simulink model "Model_6DOF_B3_2019a"  (R2019a)
settings: Solver=FixedStepAuto  StartTime=0.0  StopTime=200  FixedStep=0.05  RelTol=1e-3
values from neighbouring files (symbols this model uses):
  Ba_0 = [0 0 0 0 0 0]    [ctrl_mode_param.m]
  Bb = 4418825.3321    [load_data.m]
  Bv_0 = [tgt_speed 0 0 0 0 0]    [ctrl_mode_param.m]
  Bx_0 = [0 0 tgt_depth 0 0 0]    [ctrl_mode_param.m]
  check_angle = 10    [ctrl_mode_param.m]
  dX_imposed = 10    [ctrl_mode_param.m]
  Ixx = 5.23e7    (= 52300000)    [load_data.m]
  Ixy = 0    [load_data.m]
  Ixz = 0    [load_data.m]
  Iyy = 1.375e9    (= 1375000000)    [load_data.m]
  Iyz = 0    [load_data.m]
  Izz = 1.367e9    (= 1367000000)    [load_data.m]
  Mb = 4418825.3321    [load_data.m]
  Seastate = 5    [ctrl_mode_param.m]    (also in run.m = 0)
  Xb = 0    [load_data.m]
  Xg = 0    [load_data.m]
  Yb = 0    [load_data.m]
  Yg = 0    [load_data.m]
  Zb = 0.4406    [load_data.m]
  Zg = 0    [load_data.m]
undefined symbols (not defined in the file or in its folder): dA_BP1, dA_BP2, dA_Hull, dA_PH, dA_Sail, dA_SProot, dA_X1a, dA_X1b, dA_X2a, dA_X2b, dA_X3a, dA_X3b, dA_X4a, dA_X4b, DoF_switch, fwrite, its, LCG_switch, m_switch, mass_switch, n_BP1, n_BP2, n_Hull, n_imposed, n_PH, n_Sail, n_SProot, n_switch, n_X1a, n_X1b, n_X2a, n_X2b, n_X3a, n_X3b, n_X4a, n_X4b, nt_BP1, nt_BP2, nt_Hull, nt_PH, nt_Sail, nt_SProot, nt_X1a, nt_X1b, nt_X2a, nt_X2b, nt_X3a, nt_X3b, nt_X4a, nt_X4b, sail_switch, target_pitch, target_y, target_yaw, target_z, Usp, vt1_BP1, vt1_BP2, vt1_Hull, vt1_PH ... (+38)
libraries: simulink x5
(part 1 of 6)
settings Model: OrderedModelArguments=off  Creator=yagkim  LastModifiedBy=cooki
settings DebuggingCC: UnderSpecifiedDimensionMsg=warning

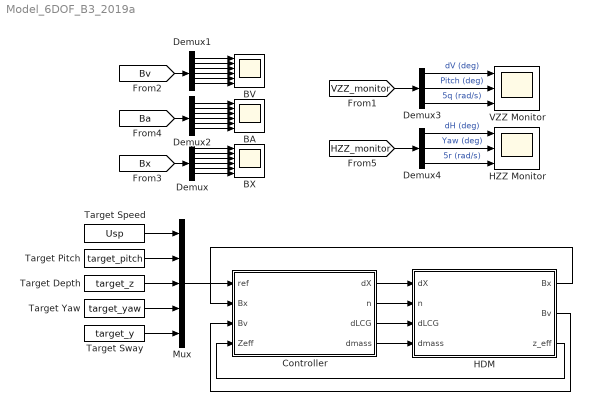
== system Model_6DOF_B3_2019a ==
  BA : Scope  NumInputPorts=6
  BV : Scope  NumInputPorts=6
  BX : Scope  NumInputPorts=6
  Controller : Subsystem
  Demux : Demux  Outputs=6
  Demux1 : Demux  Outputs=6
  Demux2 : Demux  Outputs=6
  Demux3 : Demux  Outputs=3
  Demux4 : Demux  Outputs=3
  HDM : Subsystem
  HZZ Monitor : Scope  NumInputPorts=3
  Mux : Mux  Inputs=5
  Target Depth : Constant  Value=target_z
  Target Pitch : Constant  Value=target_pitch
  Target Speed : Constant  Value=Usp
  Target Sway : Constant  Value=target_y
  Target Yaw : Constant  Value=target_yaw
  VZZ Monitor : Scope  NumInputPorts=3
  wires:
  Demux/1 -> BX/1
  Demux/2 -> BX/2
  Demux/3 -> BX/3
  Demux/6 -> BX/6
  Mux/1 -> Controller/1(ref)
  Target Speed/1 -> Mux/1
  Target Depth/1 -> Mux/3
  Demux/5 -> BX/5
  Demux2/4 -> BA/4
  Demux2/1 -> BA/1
  Demux2/3 -> BA/3
  Demux2/6 -> BA/6
  Demux2/5 -> BA/5
  Demux2/2 -> BA/2
  Target Pitch/1 -> Mux/2
  Target Yaw/1 -> Mux/4
  Target Sway/1 -> Mux/5
  Demux1/4 -> BV/4
  Demux1/6 -> BV/6
  Demux1/1 -> BV/1
  Demux1/2 -> BV/2
  Demux1/3 -> BV/3
  Demux1/5 -> BV/5
  [Bv] -> Demux1/1
  [Ba] -> Demux2/1
  [Bx] -> Demux/1
  HDM/1(Bx) -> Controller/2(Bx)
  HDM/2(Bv) -> Controller/3(Bv)
  Controller/1(dX) -> HDM/1(dX)
  Controller/2(n) -> HDM/2(n)
  Controller/3(dLCG) -> HDM/3(dLCG)
  Controller/4(dmass) -> HDM/4(dmass)
  HDM/3(z_eff) -> Controller/4(Zeff)
  Demux4/2 -> HZZ Monitor/2  "Yaw (deg)"
  [VZZ_monitor] -> Demux3/1
  Demux3/3 -> VZZ Monitor/3  "5q (rad/s)"
  Demux4/3 -> HZZ Monitor/3  "5r (rad/s)"
  Demux3/1 -> VZZ Monitor/1  "dV (deg)"
  Demux4/1 -> HZZ Monitor/1  "dH (deg)"
  [HZZ_monitor] -> Demux4/1
  Demux3/2 -> VZZ Monitor/2  "Pitch (deg)"
  Demux/4 -> BX/4

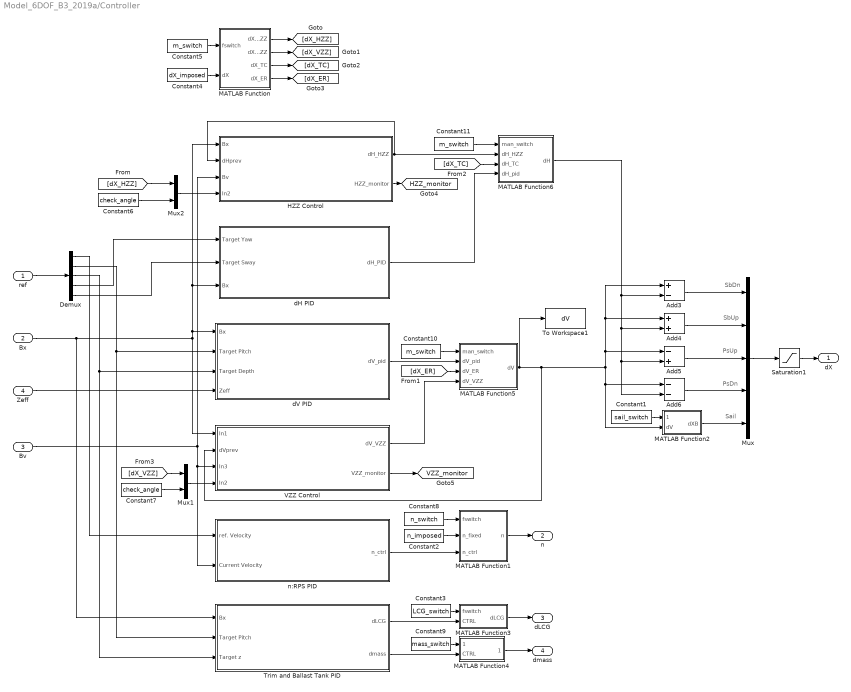
== system Model_6DOF_B3_2019a/Controller ==
  note: SbDn
  note: SbUp
  note: PsUp
  note: PsDn
  note: Sail
  ref : Inport
  Bx : Inport  Port=2
  Bv : Inport  Port=3
  Zeff : Inport  Port=4
  Add3 : Sum  Inputs=+-
  Add4 : Sum
  Add5 : Sum  Inputs=-+
  Add6 : Sum  Inputs=--
  Constant1 : Constant  Value=sail_switch
  Constant10 : Constant  Value=m_switch
  Constant11 : Constant  Value=m_switch
  Constant2 : Constant  Value=n_imposed
  Constant3 : Constant  Value=LCG_switch
  Constant4 : Constant  Value=dX_imposed
  Constant5 : Constant  Value=m_switch
  Constant6 : Constant  Value=check_angle
  Constant7 : Constant  Value=check_angle
  Constant8 : Constant  Value=n_switch
  Constant9 : Constant  Value=mass_switch
  Demux : Demux  Outputs=5
  HZZ Control : Subsystem
  MATLAB Function : MATLAB Function  TreatAsAtomicUnit=on
  MATLAB Function1 : MATLAB Function  TreatAsAtomicUnit=on
  MATLAB Function2 : MATLAB Function  TreatAsAtomicUnit=on
  MATLAB Function3 : MATLAB Function  TreatAsAtomicUnit=on
  MATLAB Function4 : MATLAB Function  TreatAsAtomicUnit=on
  MATLAB Function5 : MATLAB Function  TreatAsAtomicUnit=on
  MATLAB Function6 : MATLAB Function  TreatAsAtomicUnit=on
  Mux : Mux  Inputs=5
  Mux1 : Mux  Inputs=2
  Mux2 : Mux  Inputs=2
  Saturation1 : Saturate  UpperLimit=30  LowerLimit=-30
  To Workspace1 : ToWorkspace  VariableName=dV  SaveFormat=Timeseries  SampleTime=-1
  Trim and Ballast Tank PID : Subsystem
  VZZ Control : Subsystem
  dH PID : Subsystem
  dV PID : Subsystem
  n:RPS PID : Subsystem
  dX : Outport  VectorParamsAs1DForOutWhenUnconnected=off
  n : Outport  Port=2  VectorParamsAs1DForOutWhenUnconnected=off
  dLCG : Outport  Port=3  VectorParamsAs1DForOutWhenUnconnected=off
  dmass : Outport  Port=4  VectorParamsAs1DForOutWhenUnconnected=off
  tag scope: HZZ_monitor=global, VZZ_monitor=global
  wires:
  Add3/1 -> Mux/1
  Add4/1 -> Mux/2
  Add5/1 -> Mux/3
  Add6/1 -> Mux/4
  MATLAB Function2/1(dXB) -> Mux/5
  MATLAB Function5/1(dV) -> To Workspace1/1, VZZ Control/2(dVprev), Add3/1, Add4/1, Add5/1, MATLAB Function2/2(dV), Add6/1
  Bv/1 -> HZZ Control/3(Bv), n:RPS PID/2(Current Velocity), VZZ Control/3(In3)
  Demux/1 -> n:RPS PID/1(ref. Velocity)
  n:RPS PID/1(n_ctrl) -> MATLAB Function1/3(n_ctrl)
  ref/1 -> Demux/1
  dV PID/1(dV_pid) -> MATLAB Function5/2(dV_pid)
  Demux/4 -> dH PID/1(Target Yaw)
  Demux/5 -> dH PID/2(Target Sway)
  Mux1/1 -> VZZ Control/4(In2)
  [dX_VZZ] -> Mux1/1
  Constant7/1 -> Mux1/2
  Demux/2 -> Trim and Ballast Tank PID/2(Target Pitch), dV PID/2(Target Pitch)
  Bx/1 -> Trim and Ballast Tank PID/1(Bx), HZZ Control/1(Bx), dH PID/3(Bx), dV PID/1(Bx), VZZ Control/1(In1)
  Demux/3 -> Trim and Ballast Tank PID/3(Target z), dV PID/3(Target Depth)
  MATLAB Function3/1(dLCG) -> dLCG/1
  Mux/1 -> Saturation1/1
  Constant6/1 -> Mux2/2
  Mux2/1 -> HZZ Control/4(In2)
  [dX_HZZ] -> Mux2/1
  MATLAB Function6/1(dH) -> Add6/2, Add5/2, Add4/2, Add3/2
  Zeff/1 -> dV PID/4(Zeff)
  Saturation1/1 -> dX/1
  MATLAB Function4/1(dmass) -> dmass/1
  Constant5/1 -> MATLAB Function/1(fswitch)
  Constant4/1 -> MATLAB Function/2(dX)
  MATLAB Function/1(dX_HZZ) -> [dX_HZZ]
  MATLAB Function/2(dX_VZZ) -> [dX_VZZ]
  MATLAB Function/3(dX_TC) -> [dX_TC]
  MATLAB Function/4(dX_ER) -> [dX_ER]
  Constant8/1 -> MATLAB Function1/1(fswitch)
  Constant2/1 -> MATLAB Function1/2(n_fixed)
  MATLAB Function1/1(n) -> n/1
  Constant1/1 -> MATLAB Function2/1(fswitch)
  VZZ Control/2(VZZ_monitor) -> [VZZ_monitor]
  Trim and Ballast Tank PID/1(dLCG) -> MATLAB Function3/2(CTRL)
  Constant3/1 -> MATLAB Function3/1(fswitch)
  Trim and Ballast Tank PID/2(dmass) -> MATLAB Function4/2(CTRL)
  Constant9/1 -> MATLAB Function4/1(fswitch)
  [dX_TC] -> MATLAB Function6/3(dH_TC)
  Constant10/1 -> MATLAB Function5/1(man_switch)
  [dX_ER] -> MATLAB Function5/3(dV_ER)
  VZZ Control/1(dV_VZZ) -> MATLAB Function5/4(dV_VZZ)
  Constant11/1 -> MATLAB Function6/1(man_switch)
  HZZ Control/1(dH_HZZ) -> HZZ Control/2(dHprev), MATLAB Function6/2(dH_HZZ)
  dH PID/1(dH_PID) -> MATLAB Function6/4(dH_pid)
  HZZ Control/2(HZZ_monitor) -> [HZZ_monitor]

== system Model_6DOF_B3_2019a/HDM ==
  dX : Inport
  n : Inport  Port=2
  dLCG : Inport  Port=3
  dmass : Inport  Port=4
  Constant : Constant  Value=fwrite
  Constant1 : Constant  Value=Seastate
  HDM B3 : Subsystem  InitFcn='main'
  Integration and Coord. Transfrom : Subsystem
  Bx : Outport
  Bv : Outport  Port=2
  z_eff : Outport  Port=3
  tag scope: Ba=global, Bv=global, Bx=global
  wires:
  dLCG/1 -> HDM B3/3(dLCG)
  n/1 -> HDM B3/2(n)
  Integration and Coord. Transfrom/1(Bas) -> [Ba], HDM B3/7(Ba)
  dX/1 -> HDM B3/1(dX CTRL)
  dmass/1 -> HDM B3/4(dmass)
  HDM B3/2(z_eff) -> z_eff/1
  Integration and Coord. Transfrom/3(Bv) -> HDM B3/6(Bv), Bv/1, [Bv]
  HDM B3/1(F_hyd) -> Integration and Coord. Transfrom/2(F_hyd)
  Constant1/1 -> HDM B3/9(SeaState)
  Constant/1 -> HDM B3/8(fwrite)
  Integration and Coord. Transfrom/2("Bx ") -> Integration and Coord. Transfrom/1(Bx), HDM B3/5(Bx), Bx/1, [Bx]

== system Model_6DOF_B3_2019a/Controller/HZZ Control ==
  Bx : Inport
  dHprev : Inport  Port=2
  Bv : Inport  Port=3
  In2 : Inport  Port=4
  Clock : Clock
  Demux : Demux  Outputs=2
  Gain1 : Gain  Gain=-1
  Gain10 : Gain  Gain=180/pi
  Gain11 : Gain  Gain=5
  Gain3 : Gain
  Gain4 : Gain
  Gain8 : Gain  Gain=180/pi
  Integrator2 : Integrator
  MATLAB Function : MATLAB Function  TreatAsAtomicUnit=on
  Max Fin Rate : Constant  Value=7.11
  Mux2 : Mux  Inputs=3
  Saturation4 : Saturate  UpperLimit=20  LowerLimit=-20
  Scope : Scope
  Selector2 : Selector  InputPortWidth=6  IndexOptions=Index vector (dialog)  Indices=6  OutputSizes=1
  Selector3 : Selector  InputPortWidth=6  IndexOptions=Index vector (dialog)  Indices=6  OutputSizes=1
  dH_HZZ : Outport
  HZZ_monitor : Outport  Port=2
  wires:
  Gain11/1 -> Mux2/3
  Selector3/1 -> Gain10/1
  MATLAB Function/1(dVrate) -> Integrator2/1
  Gain10/1 -> Gain11/1
  Max Fin Rate/1 -> MATLAB Function/1(rate)
  Selector2/1 -> Gain8/1
  Clock/1 -> MATLAB Function/2(trigger)
  Gain8/1 -> Gain3/1
  Bx/1 -> Selector2/1
  Integrator2/1 -> Saturation4/1
  Saturation4/1 -> MATLAB Function/4(dVprev), Gain1/1
  Bv/1 -> Selector3/1
  Mux2/1 -> HZZ_monitor/1
  In2/1 -> Gain4/1
  Demux/1 -> MATLAB Function/5(dVmax)
  Demux/2 -> MATLAB Function/6(dXmax)
  Gain1/1 -> Scope/1, dH_HZZ/1
  Gain4/1 -> Demux/1
  Gain3/1 -> Mux2/2, MATLAB Function/3(X5)
  dHprev/1 -> Mux2/1

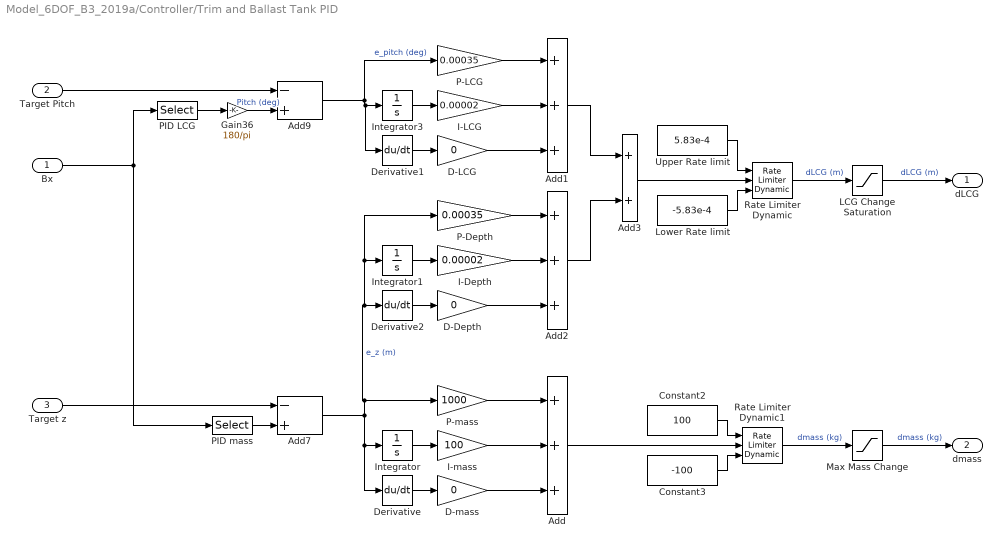
== system Model_6DOF_B3_2019a/Controller/Trim and Ballast Tank PID ==
  Bx : Inport
  Target Pitch : Inport  Port=2
  Target z : Inport  Port=3
  " LCG Change Saturation" : Saturate
  Add : Sum  Inputs=+++
  Add1 : Sum  Inputs=+++
  Add2 : Sum  Inputs=+++
  Add3 : Sum
  Add7 : Sum  Inputs=-+
  Add9 : Sum  Inputs=-+
  Constant2 : Constant  Value=100
  Constant3 : Constant  Value=-100
  D-Depth : Gain  Gain=0
  D-LCG : Gain  Gain=0
  D-mass : Gain  Gain=0
  Derivative : Derivative
  Derivative1 : Derivative
  Derivative2 : Derivative
  Gain36 : Gain  Gain=180/pi
  I-Depth : Gain  Gain=0.00002
  I-LCG : Gain  Gain=0.00002
  I-mass : Gain  Gain=100
  Integrator : Integrator
  Integrator1 : Integrator
  Integrator3 : Integrator
  Lower Rate limit : Constant  Value=-5.83e-4
  Max Mass Change : Saturate  UpperLimit=20000  LowerLimit=-20000
  P-Depth : Gain  Gain=0.00035
  P-LCG : Gain  Gain=0.00035
  P-mass : Gain  Gain=1000
  PID LCG : Selector  InputPortWidth=6  IndexOptions=Index vector (dialog)  Indices=5  OutputSizes=1
  PID mass : Selector  InputPortWidth=6  IndexOptions=Index vector (dialog)  Indices=3  OutputSizes=1
  Rate Limiter Dynamic : simulink/Discontinuities/Rate Limiter Dynamic
  Rate Limiter Dynamic1 : simulink/Discontinuities/Rate Limiter Dynamic
  Upper Rate limit : Constant  Value=5.83e-4
  dLCG : Outport
  dmass : Outport  Port=2
  wires:
  D-mass/1 -> Add/3
  Bx/1 -> PID LCG/1, PID mass/1
  I-mass/1 -> Add/2
  Gain36/1 -> Add9/2  "Pitch (deg)"
  P-LCG/1 -> Add1/1
  D-LCG/1 -> Add1/3
  PID LCG/1 -> Gain36/1
  Rate Limiter Dynamic/1 -> " LCG Change Saturation"/1  "dLCG (m)"
  Integrator/1 -> I-mass/1
  Target z/1 -> Add7/1
  Derivative/1 -> D-mass/1
  PID mass/1 -> Add7/2
  Derivative1/1 -> D-LCG/1
  Integrator3/1 -> I-LCG/1
  I-LCG/1 -> Add1/2
  P-mass/1 -> Add/1
  Target Pitch/1 -> Add9/1
  Upper Rate limit/1 -> Rate Limiter Dynamic/1
  Lower Rate limit/1 -> Rate Limiter Dynamic/3
  Max Mass Change/1 -> dmass/1  "dmass (kg)"
  Add/1 -> Rate Limiter Dynamic1/2
  Rate Limiter Dynamic1/1 -> Max Mass Change/1  "dmass (kg)"
  Constant2/1 -> Rate Limiter Dynamic1/1
  Constant3/1 -> Rate Limiter Dynamic1/3
  " LCG Change Saturation"/1 -> dLCG/1  "dLCG (m)"
  I-Depth/1 -> Add2/2
  Integrator1/1 -> I-Depth/1
  Derivative2/1 -> D-Depth/1
  D-Depth/1 -> Add2/3
  P-Depth/1 -> Add2/1
  Add3/1 -> Rate Limiter Dynamic/2
  Add1/1 -> Add3/1
  Add2/1 -> Add3/2
  Add7/1 -> Derivative/1, Integrator/1, P-Depth/1, Integrator1/1, Derivative2/1, P-mass/1  "e_z (m)"
  Add9/1 -> Derivative1/1, Integrator3/1, P-LCG/1  "e_pitch (deg)"

== system Model_6DOF_B3_2019a/Controller/VZZ Control ==
  In1 : Inport
  dVprev : Inport  Port=2
  In3 : Inport  Port=3
  In2 : Inport  Port=4
  Clock : Clock
  Demux : Demux  Outputs=2
  Gain1 : Gain  Gain=-1
  Gain10 : Gain  Gain=180/pi
  Gain11 : Gain  Gain=5
  Gain8 : Gain  Gain=180/pi
  Integrator2 : Integrator
  MATLAB Function : MATLAB Function  TreatAsAtomicUnit=on
  Max Fin Rate : Constant  Value=7.11
  Mux2 : Mux  Inputs=3
  Saturation4 : Saturate  UpperLimit=20  LowerLimit=-20
  Selector2 : Selector  InputPortWidth=6  IndexOptions=Index vector (dialog)  Indices=5  OutputSizes=1
  Selector3 : Selector  InputPortWidth=6  IndexOptions=Index vector (dialog)  Indices=5  OutputSizes=1
  dV_VZZ : Outport
  VZZ_monitor : Outport  Port=2
  wires:
  Gain11/1 -> Mux2/3
  Selector3/1 -> Gain10/1
  MATLAB Function/1(dVrate) -> Integrator2/1
  Gain10/1 -> Gain11/1
  Max Fin Rate/1 -> MATLAB Function/1(rate)
  dVprev/1 -> Mux2/1
  Selector2/1 -> Gain8/1
  Clock/1 -> MATLAB Function/2(trigger)
  Gain8/1 -> MATLAB Function/3(X5), Mux2/2
  In1/1 -> Selector2/1
  Integrator2/1 -> Saturation4/1
  Saturation4/1 -> MATLAB Function/4(dVprev), Gain1/1
  In3/1 -> Selector3/1
  Mux2/1 -> VZZ_monitor/1
  In2/1 -> Demux/1
  Demux/1 -> MATLAB Function/5(dVmax)
  Demux/2 -> MATLAB Function/6(dXmax)
  Gain1/1 -> dV_VZZ/1

== system Model_6DOF_B3_2019a/Controller/dH PID ==
  Target Yaw : Inport
  Target Sway : Inport  Port=2
  Bx : Inport  Port=3
  Add1 : Sum  Inputs=+++
  Add10 : Sum
  Add2 : Sum  Inputs=+++
  Add7 : Sum  Inputs=-+
  Add9 : Sum  Inputs=-+
  Constant : Constant  Value=7.11
  Constant1 : Constant  Value=-7.11
  D-Sway : Gain  Gain=0
  D-Yaw : Gain  Gain=12.199
  Derivative : Derivative
  Derivative1 : Derivative
  Gain36 : Gain  Gain=180/pi
  I-Sway : Gain  Gain=0
  I-Yaw : Gain  Gain=0
  Integrator : Integrator
  Integrator3 : Integrator
  Max Deflection : Saturate  UpperLimit=30  LowerLimit=-30
  P-Sway1 : Gain  Gain=-1.452
  P-Yaw : Gain  Gain=3
  PID Sway : Selector  InputPortWidth=6  IndexOptions=Index vector (dialog)  Indices=2  OutputSizes=1
  PID Yaw : Selector  InputPortWidth=6  IndexOptions=Index vector (dialog)  Indices=6  OutputSizes=1
  Rate Limiter Dynamic : simulink/Discontinuities/Rate Limiter Dynamic
  dH_PID : Outport
  wires:
  Integrator3/1 -> I-Yaw/1
  Add9/1 -> P-Yaw/1, Derivative1/1, Integrator3/1
  Add2/1 -> Add10/2
  I-Yaw/1 -> Add1/2
  Add7/1 -> P-Sway1/1, Derivative/1, Integrator/1
  Target Sway/1 -> Add7/1
  Derivative/1 -> D-Sway/1
  PID Sway/1 -> Add7/2
  P-Yaw/1 -> Add1/1
  Bx/1 -> PID Yaw/1, PID Sway/1
  I-Sway/1 -> Add2/2
  Rate Limiter Dynamic/1 -> Max Deflection/1
  D-Yaw/1 -> Add1/3
  PID Yaw/1 -> Gain36/1
  Add1/1 -> Add10/1
  Integrator/1 -> I-Sway/1
  Gain36/1 -> Add9/2
  Max Deflection/1 -> dH_PID/1
  P-Sway1/1 -> Add2/1
  D-Sway/1 -> Add2/3
  Derivative1/1 -> D-Yaw/1
  Add10/1 -> Rate Limiter Dynamic/2
  Target Yaw/1 -> Add9/1
  Constant1/1 -> Rate Limiter Dynamic/3
  Constant/1 -> Rate Limiter Dynamic/1

== system Model_6DOF_B3_2019a/Controller/dV PID ==
  Bx : Inport
  Target Pitch : Inport  Port=2
  Target Depth : Inport  Port=3
  Zeff : Inport  Port=4
  Add : Sum  Inputs=+++
  Add1 : Sum  Inputs=+++
  Add10 : Sum
  Add7 : Sum  Inputs=-+
  Add9 : Sum  Inputs=-+
  Constant : Constant  Value=7.11
  Constant1 : Constant  Value=-7.11
  D-Depth : Gain  Gain=3
  D-Pitch : Gain  Gain=3
  Derivative : Derivative
  Derivative3 : Derivative
  Gain36 : Gain  Gain=180/pi
  I-Depth : Gain  Gain=0.1044
  I-Pitch : Gain  Gain=0.1466
  I-Pitch{1..6} (6 alike) : Gain
  Integrator : Integrator
  Integrator3 : Integrator
  Max Deflection : Saturate  UpperLimit=30  LowerLimit=-30
  P-Depth : Gain  Gain=3
  P-Pitch : Gain  Gain=3
  PID Pitch : Selector  InputPortWidth=6  IndexOptions=Index vector (dialog)  Indices=5  OutputSizes=1
  Rate Limiter Dynamic : simulink/Discontinuities/Rate Limiter Dynamic
  dV_pid : Outport
  wires:
  Add/1 -> Add10/2  "dV Depth (deg)"
  Add7/1 -> Derivative3/1, Integrator/1, P-Depth/1  "Erorr in z (m)"
  Zeff/1 -> Add7/2  "z (m)"
  Integrator/1 -> I-Depth/1
  P-Depth/1 -> I-Pitch4/1
  Gain36/1 -> Add9/2  "Pitch (deg)"
  Add9/1 -> Derivative/1, Integrator3/1, P-Pitch/1  "Error in Pitch (deg)"
  P-Pitch/1 -> I-Pitch3/1
  Bx/1 -> PID Pitch/1
  Derivative3/1 -> D-Depth/1
  Add1/1 -> Add10/1  "dV Pitch (deg)"
  D-Depth/1 -> I-Pitch6/1
  Derivative/1 -> D-Pitch/1
  Integrator3/1 -> I-Pitch/1
  PID Pitch/1 -> Gain36/1
  Max Deflection/1 -> dV_pid/1  "dV"
  D-Pitch/1 -> I-Pitch5/1
  Target Pitch/1 -> Add9/1
  Add10/1 -> Rate Limiter Dynamic/2
  Rate Limiter Dynamic/1 -> Max Deflection/1
  Constant/1 -> Rate Limiter Dynamic/1
  Constant1/1 -> Rate Limiter Dynamic/3
  Target Depth/1 -> Add7/1
  I-Pitch/1 -> I-Pitch1/1
  I-Depth/1 -> I-Pitch2/1
  I-Pitch1/1 -> Add1/2
  I-Pitch2/1 -> Add/2
  I-Pitch3/1 -> Add1/1
  I-Pitch4/1 -> Add/1
  I-Pitch5/1 -> Add1/3
  I-Pitch6/1 -> Add/3

== system Model_6DOF_B3_2019a/Controller/n:RPS PID ==
  ref. Velocity : Inport
  Current Velocity : Inport  Port=2
  Add : Sum  Inputs=+++
  Add1 : Sum  Inputs=-+
  Constant1 : Constant  Value=4
  Divide : Product  Inputs=*/
  Gain1 : Gain  Gain=14.65
  Gain4 : Gain  Gain=1.465
  Integrator : Integrator
  Rate Limiter Dynamic : simulink/Discontinuities/Rate Limiter Dynamic
  Rate Max : Constant  Value=14.65
  Rate Min : Constant  Value=-14.65
  Saturation6 : Saturate  UpperLimit=10  LowerLimit=0.01
  Selector : Selector  InputPortWidth=6  IndexOptions=Index vector (dialog)  Indices=1  OutputSizes=1
  n_ctrl : Outport  VectorParamsAs1DForOutWhenUnconnected=off
  wires:
  Selector/1 -> Add1/2  "current"
  Constant1/1 -> Divide/2
  ref. Velocity/1 -> Add1/1, Divide/1  "target"
  Add1/1 -> Gain1/1, Integrator/1  "error term"
  Current Velocity/1 -> Selector/1
  Gain4/1 -> Add/3
  Gain1/1 -> Add/2
  Add/1 -> Rate Limiter Dynamic/2
  Divide/1 -> Add/1
  Rate Limiter Dynamic/1 -> Saturation6/1
  Rate Max/1 -> Rate Limiter Dynamic/1
  Rate Min/1 -> Rate Limiter Dynamic/3
  Integrator/1 -> Gain4/1
  Saturation6/1 -> n_ctrl/1

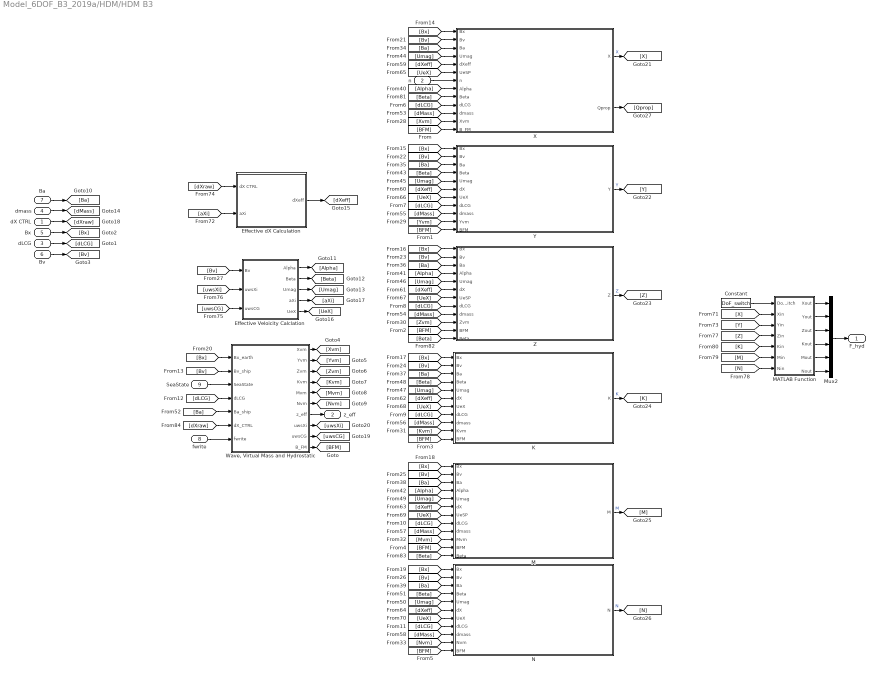
== system Model_6DOF_B3_2019a/HDM/HDM B3 ==
  dX CTRL : Inport
  n : Inport  Port=2
  dLCG : Inport  Port=3
  dmass : Inport  Port=4
  Bx : Inport  Port=5
  Bv : Inport  Port=6
  Ba : Inport  Port=7
  fwrite : Inport  Port=8
  SeaState : Inport  Port=9
  Constant : Constant  Value=DoF_switch
  Effective Veloicity Calclation : Subsystem
  Effective dX Calculation : Subsystem
  K : Subsystem
  M : Subsystem
  MATLAB Function : MATLAB Function  TreatAsAtomicUnit=on
  Mux2 : Mux  Inputs=6
  N : Subsystem
  "Wave, Virtual Mass and Hydrostatic" : Subsystem
  X : Subsystem
  Y : Subsystem
  Z : Subsystem
  F_hyd : Outport  VectorParamsAs1DForOutWhenUnconnected=off
  z_eff : Outport  Port=2  VectorParamsAs1DForOutWhenUnconnected=off
  wires:
  Mux2/1 -> F_hyd/1
  Effective dX Calculation/1(dXeff) -> [dXeff]
  Ba/1 -> [Ba]
  Bx/1 -> [Bx]
  dLCG/1 -> [dLCG]
  Bv/1 -> [Bv]
  SeaState/1 -> "Wave, Virtual Mass and Hydrostatic"/3(SeaState)
  "Wave, Virtual Mass and Hydrostatic"/7(z_eff) -> z_eff/1
  n/1 -> X/7(n)
  "Wave, Virtual Mass and Hydrostatic"/10(B_FM) -> [BFM]
  [BFM] -> X/13(B_FM)
  [BFM] -> Y/11(BFM)
  [BFM] -> Z/11(BFM)
  [BFM] -> K/11(BFM)
  [BFM] -> M/11(BFM)
  [BFM] -> N/11(BFM)
  [dLCG] -> X/10(dLCG)
  [dLCG] -> Y/8(dLCG)
  [dLCG] -> Z/8(dLCG)
  [dLCG] -> K/8(dLCG)
  [dLCG] -> M/8(dLCG)
  [dLCG] -> N/8(dLCG)
  [dLCG] -> "Wave, Virtual Mass and Hydrostatic"/4(dLCG)
  [Bx] -> X/1(Bx)
  [Bx] -> Y/1(Bx)
  [Bx] -> Z/1(Bx)
  [Bx] -> K/1(Bx)
  [Bx] -> M/1(Bx)
  [Bx] -> N/1(Bx)
  [Bx] -> "Wave, Virtual Mass and Hydrostatic"/1(Bx_earth)
  [Bv] -> "Wave, Virtual Mass and Hydrostatic"/2(Bv_ship)
  [Bv] -> X/2(Bv)
  [Bv] -> Y/2(Bv)
  [Bv] -> K/2(Bv)
  [Bv] -> M/2(Bv)
  [Bv] -> N/2(Bv)
  [Bv] -> Effective Veloicity Calclation/1(Bv)
  "Wave, Virtual Mass and Hydrostatic"/1(Xvm) -> [Xvm]
  "Wave, Virtual Mass and Hydrostatic"/2(Yvm) -> [Yvm]
  "Wave, Virtual Mass and Hydrostatic"/3(Zvm) -> [Zvm]
  "Wave, Virtual Mass and Hydrostatic"/4(Kvm) -> [Kvm]
  "Wave, Virtual Mass and Hydrostatic"/5(Mvm) -> [Mvm]
  "Wave, Virtual Mass and Hydrostatic"/6(Nvm) -> [Nvm]
  [Xvm] -> X/12(Xvm)
  [Yvm] -> Y/10(Yvm)
  [Zvm] -> Z/10(Zvm)
  [Bv] -> Z/2(Bv)
  [Kvm] -> K/10(Kvm)
  [Mvm] -> M/10(Mvm)
  [Nvm] -> N/10(Nvm)
  [Ba] -> X/3(Ba)
  [Ba] -> Y/3(Ba)
  [Ba] -> Z/3(Ba)
  [Ba] -> K/3(Ba)
  [Ba] -> M/3(Ba)
  [Ba] -> N/3(Ba)
  Effective Veloicity Calclation/1(Alpha) -> [Alpha]
  [Alpha] -> X/8(Alpha)
  [Alpha] -> Z/4(Alpha)
  [Alpha] -> M/4(Alpha)
  Effective Veloicity Calclation/2(Beta) -> [Beta]
  [Beta] -> Y/4(Beta)
  Effective Veloicity Calclation/3(Umag) -> [Umag]
  [Umag] -> X/4(Umag)
  [Umag] -> Y/5(Umag)
  [Umag] -> Z/5(Umag)
  [Umag] -> K/5(Umag)
  [Beta] -> K/4(Beta)
  [Umag] -> M/5(Umag)
  [Umag] -> N/5(Umag)
  [Beta] -> N/4(Beta)
  dmass/1 -> [dMass]
  [Ba] -> "Wave, Virtual Mass and Hydrostatic"/5(Ba_ship)
  [dMass] -> X/11(dmass)
  [dMass] -> Z/9(dmass)
  [dMass] -> Y/9(dmass)
  [dMass] -> K/9(dmass)
  [dMass] -> M/9(dmass)
  [dMass] -> N/9(dmass)
  [dXeff] -> X/5(dXeff)
  [dXeff] -> Y/6(dX)
  [dXeff] -> Z/6(dX)
  [dXeff] -> K/6(dX)
  [dXeff] -> M/6(dX)
  [dXeff] -> N/6(dX)
  Effective Veloicity Calclation/5(UeX) -> [UeX]
  [UeX] -> X/6(UeSP)
  [UeX] -> Y/7(UeX)
  [UeX] -> Z/7(UeSP)
  [UeX] -> K/7(UeX)
  [UeX] -> M/7(UeSP)
  [UeX] -> N/7(UeX)
  Effective Veloicity Calclation/4(aXi) -> [aXi]
  [aXi] -> Effective dX Calculation/2(aXi)
  dX CTRL/1 -> [dXraw]
  [dXraw] -> Effective dX Calculation/1(dX CTRL)
  "Wave, Virtual Mass and Hydrostatic"/9(uwsCG) -> [uwsCG]
  [uwsCG] -> Effective Veloicity Calclation/3(uwsCG)
  "Wave, Virtual Mass and Hydrostatic"/8(uwsXi) -> [uwsXi]
  [uwsXi] -> Effective Veloicity Calclation/2(uwsXi)
  X/1(X) -> [X]  "X"
  Y/1(Y) -> [Y]  "Y"
  Z/1(Z) -> [Z]  "Z"
  K/1(K) -> [K]  "K"
  M/1(M) -> [M]  "M"
  N/1(N) -> [N]  "N"
  [Beta] -> X/9(Beta)
  [Beta] -> Z/12(Beta)
  [Beta] -> M/12(Beta)
  [dXraw] -> "Wave, Virtual Mass and Hydrostatic"/6(dX_CTRL)
  fwrite/1 -> "Wave, Virtual Mass and Hydrostatic"/7(fwrite)
  X/2(Qprop) -> [Qprop]
  [X] -> MATLAB Function/2(Xin)
  [Y] -> MATLAB Function/3(Yin)
  [Z] -> MATLAB Function/4(Zin)
  [K] -> MATLAB Function/5(Kin)
  [M] -> MATLAB Function/6(Min)
  [N] -> MATLAB Function/7(Nin)
  Constant/1 -> MATLAB Function/1(DoF_switch)
  MATLAB Function/1(Xout) -> Mux2/1
  MATLAB Function/2(Yout) -> Mux2/2
  MATLAB Function/3(Zout) -> Mux2/3
  MATLAB Function/4(Kout) -> Mux2/4
  MATLAB Function/5(Mout) -> Mux2/5
  MATLAB Function/6(Nout) -> Mux2/6

== system Model_6DOF_B3_2019a/HDM/Integration and Coord. Transfrom ==
  Bx : Inport
  F_hyd : Inport  Port=2
  Coordinate Transform : Subsystem
  Rigid Body Motion : Subsystem
  Bas : Outport
  "Bx " : Outport  Port=2
  Bv : Outport  Port=3
  wires:
  Coordinate Transform/1(X_earth) -> "Bx "/1
  Rigid Body Motion/1(Bv) -> Bv/1, Coordinate Transform/1(Bv)
  Rigid Body Motion/2(Ba) -> Bas/1
  F_hyd/1 -> Rigid Body Motion/1(F_hyd)
  Bx/1 -> Rigid Body Motion/2(Bx)

== system Model_6DOF_B3_2019a/HDM/HDM B3/Effective Veloicity Calclation ==
  Bv : Inport
  uwsXi : Inport  Port=2
  uwsCG : Inport  Port=3
  Add{,1..4} (5 alike) : Sum
  Demux : Demux  Outputs=5
  Demux1 : Demux  Outputs=3
  Demux2 : Demux  Outputs=5
  Gain : Gain
  Gain1 : Gain
  Gain2 : Gain
  MATLAB Function : MATLAB Function  TreatAsAtomicUnit=on
  MATLAB Function1 : MATLAB Function  TreatAsAtomicUnit=on
  MATLAB Function2 : MATLAB Function  TreatAsAtomicUnit=on
  X_SP1 : Constant  Value=[31.924; 3.861; -3.861;]
  X_SP2 : Constant  Value=[31.924; 3.861; 3.861;]
  X_SP3 : Constant  Value=[31.924; -3.861; 3.861;]
  X_SP4 : Constant  Value=[31.924; -3.861; -3.861;]
  X_XB : Constant  Value=[-10.465; 0; 9.732;]
  aX : Scope  NumInputPorts=5
  n1 : Constant  Value=[0; 1/sqrt(2); -1/sqrt(2);]
  n2 : Constant  Value=[0; 1/sqrt(2); 1/sqrt(2);]
  n3 : Constant  Value=[0; -1/sqrt(2); 1/sqrt(2);]
  n4 : Constant  Value=[0; -1/sqrt(2); -1/sqrt(2);]
  n5 : Constant  Value=[0; 1; 0;]
  nh : Constant  Value=[-1; 0; 0;]
  urXi : Scope  NumInputPorts=5
  Alpha : Outport
  Beta : Outport  Port=2
  Umag : Outport  Port=3
  aXi : Outport  Port=4
  UeX : Outport  Port=5
  wires:
  Bv/1 -> MATLAB Function1/6(U_ship), MATLAB Function2/1(Bv)
  nh/1 -> MATLAB Function/1(nh)
  n1/1 -> MATLAB Function/2(n1)
  n2/1 -> MATLAB Function/3(n2)
  n3/1 -> MATLAB Function/4(n3)
  n4/1 -> MATLAB Function/5(n4)
  X_XB/1 -> MATLAB Function1/5(rXB)
  X_SP2/1 -> MATLAB Function1/2(rX2)
  X_SP3/1 -> MATLAB Function1/3(rX3)
  X_SP4/1 -> MATLAB Function1/4(rX4)
  X_SP1/1 -> MATLAB Function1/1(rX1)
  n5/1 -> MATLAB Function/6(nB)
  MATLAB Function1/1(urX1) -> Add/1, urXi/1
  MATLAB Function/1(aX) -> Gain1/1, Demux2/1
  Demux/1 -> Add/2
  Add/1 -> MATLAB Function/7(urX1)
  Add1/1 -> MATLAB Function/8(urX2)
  Add2/1 -> MATLAB Function/9(urX3)
  Add3/1 -> MATLAB Function/10(urX4)
  Add4/1 -> MATLAB Function/11(urXB)
  Demux/2 -> Add1/2
  Demux/3 -> Add2/2
  Demux/4 -> Add3/2
  Demux/5 -> Add4/2
  MATLAB Function1/5(urXB) -> Add4/1, urXi/5
  MATLAB Function1/4(urX4) -> Add3/1, urXi/4
  MATLAB Function1/3(urX3) -> Add2/1, urXi/3
  MATLAB Function1/2(urX2) -> Add1/1, urXi/2
  MATLAB Function2/1(alpha) -> Gain/1
  MATLAB Function2/2(beta) -> Beta/1
  MATLAB Function2/3(Umag) -> Umag/1
  MATLAB Function/2(UeX) -> UeX/1
  Demux1/1 -> MATLAB Function2/2(uCG)
  Demux1/2 -> MATLAB Function2/3(vCG)
  Demux1/3 -> MATLAB Function2/4(wCG)
  Demux2/1 -> aX/1
  Demux2/2 -> aX/2
  Demux2/3 -> aX/3
  Demux2/4 -> aX/4
  Demux2/5 -> aX/5
  uwsCG/1 -> Demux1/1
  Gain/1 -> Alpha/1
  Gain1/1 -> aXi/1
  Gain2/1 -> Demux/1
  uwsXi/1 -> Gain2/1

== system Model_6DOF_B3_2019a/HDM/HDM B3/Effective dX Calculation ==
  dX CTRL : Inport
  aXi : Inport  Port=2
  Add{,1..4} (5 alike) : Sum
  Demux : Demux  Outputs=5
  Demux1 : Demux  Outputs=5
  Mux6 : Mux  Inputs=5
  dXeff : Outport
  wires:
  dX CTRL/1 -> Demux/1
  aXi/1 -> Demux1/1
  Add/1 -> Mux6/1
  Add1/1 -> Mux6/2
  Add2/1 -> Mux6/3
  Add3/1 -> Mux6/4
  Add4/1 -> Mux6/5
  Demux/1 -> Add/1
  Demux/2 -> Add1/1
  Demux/3 -> Add2/1
  Demux/4 -> Add3/1
  Demux/5 -> Add4/1
  Demux1/1 -> Add/2
  Demux1/2 -> Add1/2
  Demux1/3 -> Add2/2
  Demux1/4 -> Add3/2
  Demux1/5 -> Add4/2
  Mux6/1 -> dXeff/1

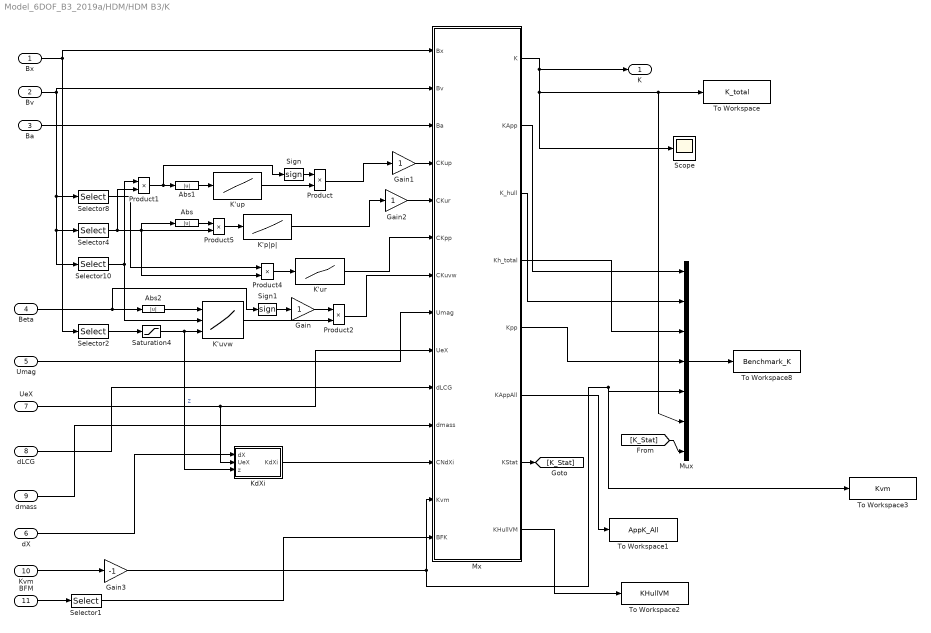
== system Model_6DOF_B3_2019a/HDM/HDM B3/K ==
  Bx : Inport
  Bv : Inport  Port=2
  Ba : Inport  Port=3
  Beta : Inport  Port=4
  Umag : Inport  Port=5
  dX : Inport  Port=6
  UeX : Inport  Port=7
  dLCG : Inport  Port=8
  dmass : Inport  Port=9
  Kvm : Inport  Port=10
  BFM : Inport  Port=11
  Abs : Abs
  Abs1 : Abs
  Abs2 : Abs
  Gain : Gain
  Gain1 : Gain
  Gain2 : Gain
  Gain3 : Gain  Gain=-1
  K'p|p| : Lookup_n-D  NumberOfTableDimensions=1  BreakpointsForDimension1=|  Table=|  InternalRulePriority=Speed  RndMeth=Simplest  InputSameDT=on
      BreakpointsForDimension1=|
      | [-0.0015
      | -0.0012
      | -0.0009
      | -0.0006
      | -0.0003
      | -0.0001
      | 0.0001
      | 0.0003
      | 0.0006
      | 0.0009
      | 0.0012
      | 0.0015]
      Table=|
      | [-1.3011E-02
      | -1.6962E-02
      | -2.0682E-02
      | -3.1419E-02
      | -6.4407E-02
      | -1.9322E-01
      | 1.9322E-01
      | 6.4378E-02
      | 3.1944E-02
      | 2.1072E-02
      | 1.6415E-02
      | 1.3407E-02]
  K'up : Lookup_n-D  NumberOfTableDimensions=1  BreakpointsForDimension1=|  Table=|  InternalRulePriority=Speed  RndMeth=Simplest  InputSameDT=on
      BreakpointsForDimension1=|
      | [0.03999989
      | 0.079999993
      | 0.11999963
      | 0.15999956]
      Table=|
      | [-4.0344E-04
      | -8.1402E-04
      | -1.2116E-03
      | -1.6125E-03]
  K'ur : Lookup_n-D  NumberOfTableDimensions=1  BreakpointsForDimension1=|  Table=|  InternalRulePriority=Speed  RndMeth=Simplest  InputSameDT=on
      BreakpointsForDimension1=|
      | [-0.0015
      | -0.0012
      | -0.0009
      | -0.0006
      | -0.0003
      | -0.0001
      | 0.0001
      | 0.0003
      | 0.0006
      | 0.0009
      | 0.0012
      | 0.0015]
      Table=|
      | [-1.3011E-02
      | -1.6962E-02
      | -2.0682E-02
      | -3.1419E-02
      | -6.4407E-02
      | -1.9322E-01
      | 1.9322E-01
      | 6.4378E-02
      | 3.1944E-02
      | 2.1072E-02
      | 1.6415E-02
      | 1.3407E-02]
  K'uvw : Lookup_n-D  NumberOfTableDimensions=3  BreakpointsForDimension1=|  BreakpointsForDimension2=|  BreakpointsForDimension3=|  Table=|  InternalRulePriority=Speed  RndMeth=Simplest  InputSameDT=on
      BreakpointsForDimension1=|
      | [0
      | 4
      | 8
      | 12]
      BreakpointsForDimension2=|
      | [-5.1444E+00
      | -3.0866E+00
      | -1.5433E+00
      | ]
      Table=|
      | reshape([0.0000000E+00
      | 1.5570290E-04
      | 3.7677829E-04
      | 6.0025374E-04
      | 0.0000000E+00
      | 1.5575678E-04
      | 3.8557685E-04
      | 6.0103850E-04
      | 0.0000000E+00
      | 1.7511088E-04
      | 3.8376789E-04
      | 6.0108480E-04
      | 0.0000000E+00
      | 1.9071552E-04
      | 4.0986649E-04
      | 6.4012030E-04
      | 0.0000000E+00
      | 1.8940622E-04
      | 4.0946931E-04
      | 6.3613461E-04
      | 0.0000000E+00
      | 1.8621071E-04
      | 4.0619654E-04
      | 7.0286379E-04
      | 0.0000000E+00
      | 2.0712189E-04
      | 4.4751988E-04
      | 7.0514631E-04
      | 0.0000000E+00
      | 1.9895751E-04
      | 4.3099356E-04
      | 6.6994571E-04
      | 0.0000000E+00
      | 1.9568554E-04
      | 4.2679977E-04
      | 6.6445067E-04
      | 0.0000000E+00
      | 2.4359563E-04
      | 5.3740096E-04
      | 8.5879902E-04
      | 0.0000000E+00
      | 2.0890025E-04
      | 4.5502130E-04
      | 7.1388224E-04
      | 0.0000000E+00
      | 2.0575072E-04
      | 4.5505766E-04
      | 7.0285206E-04],[4,3,4])
      BreakpointsForDimension3=|
      | [-35.0624 -18.3724 -15.3724 -13.8724
      | ]
  KdXi : Subsystem
  Mux : Mux  Inputs=7
  Mx : MATLAB Function  TreatAsAtomicUnit=on
  Product{,1..2,4..5} (5 alike) : Product
  Saturation4 : Saturate  UpperLimit=-13.8724  LowerLimit=-35.0624
  Scope : Scope
  Selector1 : Selector  InputPortWidth=6  IndexOptions=Index vector (dialog)  Indices=4  OutputSizes=1
  Selector10 : Selector  InputPortWidth=6  IndexOptions=Index vector (dialog)  Indices=1  OutputSizes=1
  Selector2 : Selector  InputPortWidth=6  IndexOptions=Index vector (dialog)  Indices=3  OutputSizes=1
  Selector4 : Selector  InputPortWidth=6  IndexOptions=Index vector (dialog)  Indices=4  OutputSizes=1
  Selector8 : Selector  InputPortWidth=6  IndexOptions=Index vector (dialog)  Indices=2  OutputSizes=1
  Sign : Signum
  Sign1 : Signum
  To Workspace : ToWorkspace  VariableName=K_total  SaveFormat=Timeseries  SampleTime=-1
  To Workspace1 : ToWorkspace  VariableName=AppK_All  SaveFormat=Timeseries  SampleTime=-1
  To Workspace2 : ToWorkspace  VariableName=KHullVM  SaveFormat=Timeseries  SampleTime=-1
  To Workspace3 : ToWorkspace  VariableName=Kvm  SaveFormat=Timeseries  SampleTime=-1
  To Workspace8 : ToWorkspace  VariableName=Benchmark_K  SaveFormat=Timeseries  SampleTime=-1
  K : Outport
  wires:
  Bv/1 -> Selector10/1, Selector4/1, Selector8/1, Mx/2(Bv)
  Bx/1 -> Mx/1(Bx), Selector2/1
  Selector10/1 -> K'uvw/2, Product1/1
  Ba/1 -> Mx/3(Ba)
  UeX/1 -> KdXi/2(UeX), Mx/9(UeX)
  Beta/1 -> Sign1/1, Abs2/1
  Umag/1 -> Mx/8(Umag)
  dLCG/1 -> Mx/10(dLCG)
  dmass/1 -> Mx/11(dmass)
  dX/1 -> KdXi/1(dX)
  K'up/1 -> Product/2
  K'p|p|/1 -> Gain2/1
  Product4/1 -> K'ur/1
  Selector8/1 -> Product4/1
  Abs/1 -> Product5/1
  Product5/1 -> K'p|p|/1
  Selector4/1 -> Product1/2, Product5/2, Abs/1, Product4/2
  K'ur/1 -> Mx/6(CKpp)
  KdXi/1(KdXi) -> Mx/12(CNdXi)
  Selector2/1 -> Saturation4/1
  K'uvw/1 -> Product2/2
  Product1/1 -> Sign/1, Abs1/1
  Abs1/1 -> K'up/1
  Sign/1 -> Product/1
  Product/1 -> Gain1/1
  Product2/1 -> Mx/7(CKuvw)
  Abs2/1 -> K'uvw/1
  Sign1/1 -> Gain/1
  Mux/1 -> To Workspace8/1
  Mx/2(KApp) -> Mux/1
  Mx/3(K_hull) -> Mux/2
  Mx/4(Kh_total) -> Mux/3
  Mx/5(Kpp) -> Mux/4
  Mx/6(KAppAll) -> To Workspace1/1
  BFM/1 -> Selector1/1
  Selector1/1 -> Mx/14(BFK)
  Mx/1(K) -> Scope/1, Mux/6, To Workspace/1, K/1
  Mx/7(KStat) -> [K_Stat]
  Gain/1 -> Product2/1
  Gain1/1 -> Mx/4(CKup)
  Gain2/1 -> Mx/5(CKur)
  [K_Stat] -> Mux/7
  Saturation4/1 -> KdXi/3(z), K'uvw/3  "z"
  Mx/8(KHullVM) -> To Workspace2/1
  Kvm/1 -> Gain3/1
  Gain3/1 -> Mx/13(Kvm), To Workspace3/1, Mux/5

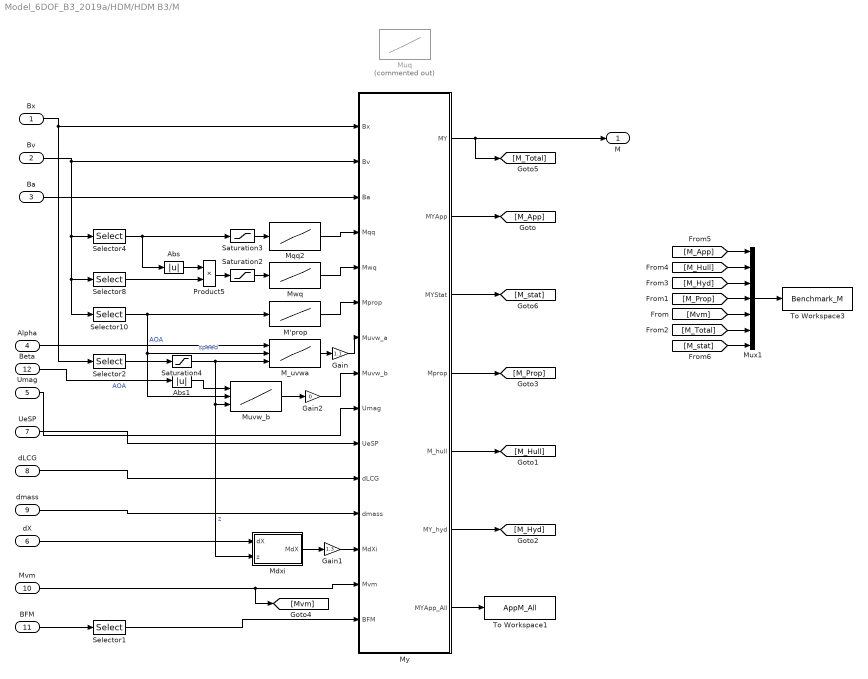
== system Model_6DOF_B3_2019a/HDM/HDM B3/M ==
  Bx : Inport
  Bv : Inport  Port=2
  Ba : Inport  Port=3
  Alpha : Inport  Port=4
  Umag : Inport  Port=5
  dX : Inport  Port=6
  UeSP : Inport  Port=7
  dLCG : Inport  Port=8
  dmass : Inport  Port=9
  Mvm : Inport  Port=10
  BFM : Inport  Port=11
  Beta : Inport  Port=12
  Abs : Abs
  Abs1 : Abs
  Gain : Gain  Gain=1.1
  Gain1 : Gain  Gain=1.3
  Gain2 : Gain  Gain=0
  M'prop : Lookup_n-D  NumberOfTableDimensions=1  BreakpointsForDimension1=[-7.7166666 -5.1444444 -3.08666664]  Table=[-0.00022 -0.0002 -0.00015]  InternalRulePriority=Speed  RndMeth=Simplest  InputSameDT=on
  M_uvwa : Lookup_n-D  NumberOfTableDimensions=3  BreakpointsForDimension1=|  BreakpointsForDimension2=|  BreakpointsForDimension3=|  Table=|  InternalRulePriority=Speed  RndMeth=Simplest  InputSameDT=on
      BreakpointsForDimension1=|
      | [-12
      | -8
      | -4
      | 0
      | 4
      | 8
      | 12]
      BreakpointsForDimension2=|
      | [-5.1444E+00
      | -3.0866E+00
      | -1.5433E+00
      | ]
      Table=|
      | reshape([-2.40251E-03
      | -1.59538E-03
      | -8.21748E-04
      | -3.60182E-06
      | 8.13350E-04
      | 1.50586E-03
      | 2.39707E-03
      | -2.43392E-03
      | -1.61509E-03
      | -8.50748E-04
      | -3.60182E-06
      | 8.24271E-04
      | 1.51842E-03
      | 2.43805E-03
      | -2.45014E-03
      | -1.65711E-03
      | -9.11210E-04
      | -3.60182E-06
      | 8.61300E-04
      | 1.57459E-03
      | 2.42777E-03
      | -2.54380E-03
      | -1.68842E-03
      | -8.33041E-04
      | 2.23377E-05
      | 8.77717E-04
      | 1.73310E-03
      | 2.58847E-03
      | -2.63734E-03
      | -1.75078E-03
      | -8.64221E-04
      | 2.23377E-05
      | 9.08896E-04
      | 1.79546E-03
      | 2.68201E-03
      | -2.83738E-03
      | -1.88414E-03
      | -9.30902E-04
      | 2.23377E-05
      | 9.75577E-04
      | 1.92882E-03
      | 2.88206E-03
      | -2.63786E-03
      | -1.74504E-03
      | -8.52211E-04
      | 4.06140E-05
      | 9.33439E-04
      | 1.82626E-03
      | 2.71909E-03
      | -2.63728E-03
      | -1.74465E-03
      | -8.52017E-04
      | 4.06140E-05
      | 9.33245E-04
      | 1.82588E-03
      | 2.71851E-03
      | -2.86138E-03
      | -1.89405E-03
      | -9.26716E-04
      | 4.06140E-05
      | 1.00794E-03
      | 1.97527E-03
      | 2.94260E-03
      | -0.002723494
      | -0.001792522
      | -0.000861549
      | 6.9423E-05
      | 0.001000396
      | 0.001931368
      | 0.002862341
      | -0.002736476
      | -0.001798489
      | -0.000860502
      | 6.9423E-05
      | 0.001015473
      | 0.00195346
      | 0.002891447
      | -0.002765582
      | -0.00182058
      | -0.000875579
      | 6.9423E-05
      | 0.001014425
      | 0.001959426
      | 0.002904428],[7,3,4])
      BreakpointsForDimension3=|
      | [-35.0624 -18.3724 -15.3724 -13.8724
      | ]
  Mdxi : Subsystem
  Mqq2 : Lookup_n-D  NumberOfTableDimensions=1  BreakpointsForDimension1=|  Table=|  InternalRulePriority=Speed  RndMeth=Simplest  InputSameDT=on
      BreakpointsForDimension1=|
      | [-0.02
      | -0.015
      | -0.012958963
      | -0.009719222
      | -0.006479482
      | -0.003239741
      | -0.00161987
      | -0.000647948
      | 0.000647948
      | 0.00161987
      | 0.003239741
      | 0.006479482
      | 0.009719222
      | 0.012958963
      | 0.015
      | 0.02
      | ]
      Table=|
      | [-2.2571E-03
      | -2.3029E-03
      | -2.0965E-03
      | -2.0229E-03
      | -2.1546E-03
      | -1.4789E-03
      | -1.5664E-03
      | -1.4544E-03
      | -1.4705E-03
      | -1.4942E-03
      | -1.8790E-03
      | -1.8821E-03
      | -2.1009E-03
      | -2.0521E-03
      | -2.1685E-03
      | -2.0822E-03
      | ]
  Muq : Lookup_n-D  Commented=on  BreakpointsForDimension1=|  BreakpointsForDimension2=|  Table=|  InternalRulePriority=Speed  RndMeth=Simplest  InputSameDT=on
      BreakpointsForDimension1=|
      | [-2.00E-01
      | -1.50E-01
      | -1.00E-01
      | -5.00E-02
      | 0.00E+00
      | 5.00E-02
      | 1.00E-01
      | 1.50E-01
      | 2.00E-01
      | ]
      Table=|
      | reshape([-3.95902E-04
      | -2.96922E-04
      | -1.97952E-04
      | -9.89720E-05
      | 0.00000E+00
      | 9.89750E-05
      | 1.97948E-04
      | 2.96928E-04
      | 3.95898E-04
      | -4.94864E-04
      | -3.71144E-04
      | -2.47434E-04
      | -1.23714E-04
      | 0.00000E+00
      | 1.23715E-04
      | 2.47426E-04
      | 3.71146E-04
      | 4.94856E-04
      | -5.69298E-04
      | -4.26978E-04
      | -2.84648E-04
      | -1.42328E-04
      | 0.00000E+00
      | 1.42322E-04
      | 2.84652E-04
      | 4.26972E-04
      | 5.69302E-04
      | -5.60922E-04
      | -4.20692E-04
      | -2.80462E-04
      | -1.40232E-04
      | 0.00000E+00
      | 1.40228E-04
      | 2.80458E-04
      | 4.20688E-04
      | 5.60918E-04],[9,4])
      BreakpointsForDimension2=|
      | [-7.7166 -5.1444 -3.08664 -1.54332
      | ]
  Muvw_b : Lookup_n-D  NumberOfTableDimensions=3  BreakpointsForDimension1=|  BreakpointsForDimension2=|  BreakpointsForDimension3=|  Table=|  InternalRulePriority=Speed  RndMeth=Simplest  InputSameDT=on
      BreakpointsForDimension1=|
      | [0
      | 4
      | 8
      | 12]
      BreakpointsForDimension2=|
      | [-5.1444E+00
      | -3.0866E+00
      | -1.5433E+00
      | ]
      Table=|
      | reshape([0.0000000E+00
      | 1.7951756E-04
      | 5.3168107E-04
      | 8.2196049E-04
      | 0.0000000E+00
      | 1.8161260E-04
      | 4.0651122E-04
      | 8.4309870E-04
      | 0.0000000E+00
      | 1.5982719E-04
      | 3.9808975E-04
      | 8.3394733E-04
      | 0.0000000E+00
      | 1.6730861E-04
      | 4.2653453E-04
      | 8.8590611E-04
      | 0.0000000E+00
      | 1.7226773E-04
      | 4.2301121E-04
      | 9.1415390E-04
      | 0.0000000E+00
      | 1.7161548E-04
      | 4.4496312E-04
      | 1.0670148E-03
      | 0.0000000E+00
      | 1.8499821E-04
      | 4.5439059E-04
      | 1.0035581E-03
      | 0.0000000E+00
      | 1.8604595E-04
      | 4.6158821E-04
      | 9.9911572E-04
      | 0.0000000E+00
      | 1.8299862E-04
      | 4.6898472E-04
      | 9.8070400E-04
      | 0.0000000E+00
      | 2.0633449E-04
      | 5.3479606E-04
      | 1.1592712E-03
      | 0.0000000E+00
      | 1.9483340E-04
      | 4.8156088E-04
      | 1.0722724E-03
      | 0.0000000E+00
      | 1.8941258E-04
      | 4.6648371E-04
      | 1.0463937E-03],[4,3,4])
      BreakpointsForDimension3=|
      | [-35.0624 -18.3724 -15.3724 -13.8724
      | ]
  Mux1 : Mux  Inputs=7
  Mwq : Lookup_n-D  NumberOfTableDimensions=1  BreakpointsForDimension1=|  Table=|  InternalRulePriority=Speed  RndMeth=Simplest  InputSameDT=on
      BreakpointsForDimension1=|
      | [-0.0015
      | -0.0012
      | -0.0009
      | -0.0006
      | -0.0003
      | -0.0001
      | 0.0001
      | 0.0003
      | 0.0006
      | 0.0009
      | 0.0012
      | 0.0015]
      Table=|
      | [-1.3011E-02
      | -1.6962E-02
      | -2.0682E-02
      | -3.1419E-02
      | -6.4407E-02
      | -1.9322E-01
      | 1.9322E-01
      | 6.4378E-02
      | 3.1944E-02
      | 2.1072E-02
      | 1.6415E-02
      | 1.3407E-02]
  My : MATLAB Function  TreatAsAtomicUnit=on
  Product5 : Product
  Saturation2 : Saturate  UpperLimit=0.0015  LowerLimit=-0.0015
  Saturation3 : Saturate  UpperLimit=0.02  LowerLimit=-0.02
  Saturation4 : Saturate  UpperLimit=-13.8724  LowerLimit=-35.0624
  Selector1 : Selector  InputPortWidth=6  IndexOptions=Index vector (dialog)  Indices=5  OutputSizes=1
  Selector10 : Selector  InputPortWidth=6  IndexOptions=Index vector (dialog)  Indices=1  OutputSizes=1
  Selector2 : Selector  InputPortWidth=6  IndexOptions=Index vector (dialog)  Indices=3  OutputSizes=1
  Selector4 : Selector  InputPortWidth=6  IndexOptions=Index vector (dialog)  Indices=5  OutputSizes=1
  Selector8 : Selector  InputPortWidth=6  IndexOptions=Index vector (dialog)  Indices=3  OutputSizes=1
  To Workspace1 : ToWorkspace  VariableName=AppM_All  SaveFormat=Timeseries  SampleTime=-1
  To Workspace3 : ToWorkspace  VariableName=Benchmark_M  SaveFormat=Timeseries  SampleTime=-1
  M : Outport
  wires:
  M_uvwa/1 -> Gain/1
  Selector2/1 -> Saturation4/1
  Mvm/1 -> My/14(Mvm), [Mvm]
  Mdxi/1(MdX) -> Gain1/1
  My/1(MY) -> M/1, [M_Total]
  Saturation3/1 -> Mqq2/1
  Saturation2/1 -> Mwq/1
  Abs/1 -> Product5/1
  Selector8/1 -> Product5/2
  Product5/1 -> Saturation2/1
  Mwq/1 -> My/5(Mwq)
  Mqq2/1 -> My/4(Mqq)
  dX/1 -> Mdxi/1(dX)
  dmass/1 -> My/12(dmass)
  dLCG/1 -> My/11(dLCG)
  Umag/1 -> My/9(Umag)
  Alpha/1 -> M_uvwa/1  "AOA"
  Selector4/1 -> Abs/1, Saturation3/1
  UeSP/1 -> My/10(UeSP)
  M'prop/1 -> My/6("Mprop ")
  Ba/1 -> My/3(Ba)
  Selector10/1 -> M_uvwa/2, Muvw_b/2, M'prop/1  "speed"
  Bx/1 -> My/1(Bx), Selector2/1
  Bv/1 -> Selector10/1, Selector8/1, Selector4/1, My/2(Bv)
  My/3(MYStat) -> [M_stat]
  Saturation4/1 -> Mdxi/2(z), Muvw_b/3, M_uvwa/3  "z"
  Gain/1 -> My/7(Muvw_a)
  My/7(MYApp_All) -> To Workspace1/1
  BFM/1 -> Selector1/1
  Selector1/1 -> My/15(BFM)
  [Mvm] -> Mux1/5
  [M_Prop] -> Mux1/4
  [M_App] -> Mux1/1
  [M_Hyd] -> Mux1/3
  Mux1/1 -> To Workspace3/1
  [M_Hull] -> Mux1/2
  [M_Total] -> Mux1/6
  My/2(MYApp) -> [M_App]
  My/5(M_hull) -> [M_Hull]
  My/6(MY_hyd) -> [M_Hyd]
  My/4(Mprop) -> [M_Prop]
  Gain1/1 -> My/13(MdXi)
  [M_stat] -> Mux1/7
  Muvw_b/1 -> Gain2/1
  Beta/1 -> Abs1/1  "AOA"
  Abs1/1 -> Muvw_b/1
  Gain2/1 -> My/8(Muvw_b)

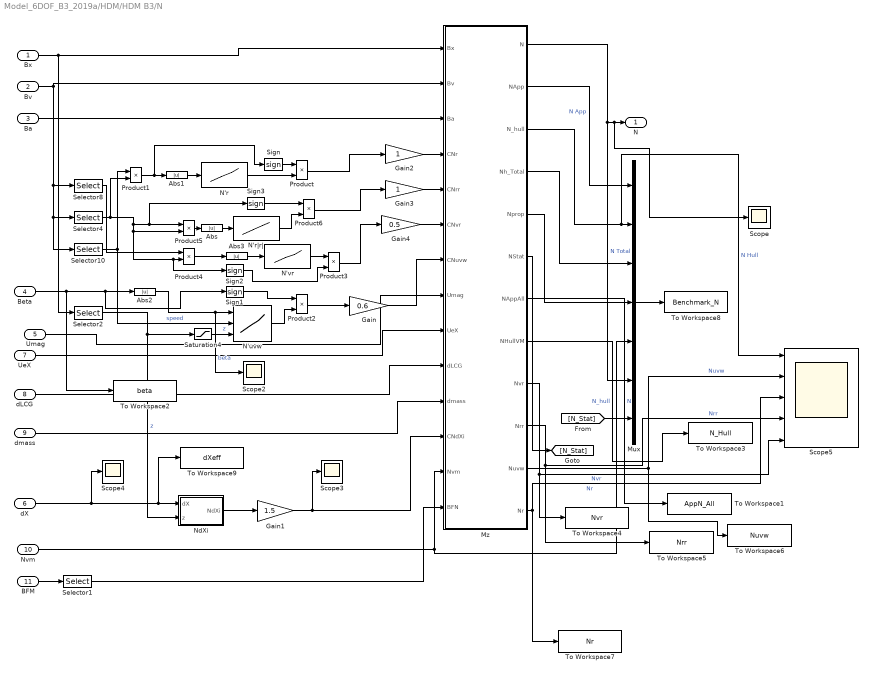
== system Model_6DOF_B3_2019a/HDM/HDM B3/N ==
  Bx : Inport
  Bv : Inport  Port=2
  Ba : Inport  Port=3
  Beta : Inport  Port=4
  Umag : Inport  Port=5
  dX : Inport  Port=6
  UeX : Inport  Port=7
  dLCG : Inport  Port=8
  dmass : Inport  Port=9
  Nvm : Inport  Port=10
  BFM : Inport  Port=11
  Abs{,1..3} (4 alike) : Abs
  Gain : Gain  Gain=0.6
  Gain1 : Gain  Gain=1.5
  Gain2 : Gain
  Gain3 : Gain
  Gain4 : Gain  Gain=0.5
  Mux : Mux  Inputs=7
  Mz : MATLAB Function  TreatAsAtomicUnit=on
  N'r : Lookup_n-D  NumberOfTableDimensions=1  BreakpointsForDimension1=|  Table=|  InternalRulePriority=Speed  RndMeth=Simplest  InputSameDT=on
      BreakpointsForDimension1=|
      | [0.03999989
      | 0.079999993
      | 0.11999963
      | 0.15999956]
      Table=|
      | [-4.0344E-04
      | -8.1402E-04
      | -1.2116E-03
      | -1.6125E-03]
  N'r|r| : Lookup_n-D  NumberOfTableDimensions=1  BreakpointsForDimension1=|  Table=|  InternalRulePriority=Speed  RndMeth=Simplest  InputSameDT=on
      BreakpointsForDimension1=|
      | [0.0001
      | 0.0003
      | 0.0006
      | 0.0009
      | 0.0012
      | 0.0015
      | ]
      Table=|
      | [1.93E-01
      | 6.44E-02
      | 3.19E-02
      | 2.11E-02
      | 1.64E-02
      | 1.34E-02
      | ]
  N'uvw : Lookup_n-D  NumberOfTableDimensions=3  BreakpointsForDimension1=|  BreakpointsForDimension2=|  BreakpointsForDimension3=|  Table=|  InternalRulePriority=Speed  RndMeth=Simplest  InputSameDT=on
      BreakpointsForDimension1=|
      | [0
      | 4
      | 8
      | 12]
      BreakpointsForDimension2=|
      | [-5.1444E+00
      | -3.0866E+00
      | -1.5433E+00
      | ]
      Table=|
      | reshape([0.0000000E+00
      | 1.1975814E-03
      | 2.7970643E-03
      | 4.1308534E-03
      | 0.0000000E+00
      | 1.2111628E-03
      | 2.9207146E-03
      | 4.1207837E-03
      | 0.0000000E+00
      | 1.4959851E-03
      | 2.9486406E-03
      | 4.1213058E-03
      | 0.0000000E+00
      | 1.4879743E-03
      | 2.9975710E-03
      | 4.2577903E-03
      | 0.0000000E+00
      | 1.4933232E-03
      | 3.0017417E-03
      | 4.2334501E-03
      | 0.0000000E+00
      | 1.5365285E-03
      | 3.0446384E-03
      | 4.4091424E-03
      | 0.0000000E+00
      | 1.5329300E-03
      | 3.0664177E-03
      | 4.3937198E-03
      | 0.0000000E+00
      | 1.5274021E-03
      | 3.0742094E-03
      | 4.3066710E-03
      | 0.0000000E+00
      | 1.5692494E-03
      | 3.1052278E-03
      | 4.3211963E-03
      | 0.0000000E+00
      | 1.5996020E-03
      | 3.2227652E-03
      | 4.5425478E-03
      | 0.0000000E+00
      | 1.5650123E-03
      | 3.1236229E-03
      | 4.4022471E-03
      | 0.0000000E+00
      | 1.6041810E-03
      | 3.1241151E-03
      | 4.4103656E-03],[4,3,4])
      BreakpointsForDimension3=|
      | [-35.0624 -18.3724 -15.3724 -13.8724
      | ]
  N'vr : Lookup_n-D  NumberOfTableDimensions=1  BreakpointsForDimension1=|  Table=|  InternalRulePriority=Speed  RndMeth=Simplest  InputSameDT=on
      BreakpointsForDimension1=|
      | [0
      | 0.051444
      | 0.102888
      | 0.205776
      | 0.411552]
      Table=|
      | [0.0000E+00
      | -1.9921E-03
      | -9.2025E-03
      | -3.2154E-02
      | -1.3255E-01]
  NdXi : Subsystem
  Product{,1..6} (7 alike) : Product
  Saturation4 : Saturate  UpperLimit=-13.8724  LowerLimit=-35.0624
  Scope{,2..4} (4 alike) : Scope
  Scope5 : Scope  NumInputPorts=5
  Selector1 : Selector  InputPortWidth=6  IndexOptions=Index vector (dialog)  Indices=6  OutputSizes=1
  Selector10 : Selector  InputPortWidth=6  IndexOptions=Index vector (dialog)  Indices=1  OutputSizes=1
  Selector2 : Selector  InputPortWidth=6  IndexOptions=Index vector (dialog)  Indices=3  OutputSizes=1
  Selector4 : Selector  InputPortWidth=6  IndexOptions=Index vector (dialog)  Indices=6  OutputSizes=1
  Selector8 : Selector  InputPortWidth=6  IndexOptions=Index vector (dialog)  Indices=2  OutputSizes=1
  Sign{,1..3} (4 alike) : Signum
  To Workspace1 : ToWorkspace  VariableName=AppN_All  SaveFormat=Timeseries  SampleTime=-1
  To Workspace2 : ToWorkspace  VariableName=beta  SaveFormat=Timeseries  SampleTime=-1
  To Workspace3 : ToWorkspace  VariableName=N_Hull  SaveFormat=Timeseries  SampleTime=-1
  To Workspace4 : ToWorkspace  VariableName=Nvr  SaveFormat=Timeseries  SampleTime=-1
  To Workspace5 : ToWorkspace  VariableName=Nrr  SaveFormat=Timeseries  SampleTime=-1
  To Workspace6 : ToWorkspace  VariableName=Nuvw  SaveFormat=Timeseries  SampleTime=-1
  To Workspace7 : ToWorkspace  VariableName=Nr  SaveFormat=Timeseries  SampleTime=-1
  To Workspace8 : ToWorkspace  VariableName=Benchmark_N  SaveFormat=Timeseries  SampleTime=-1
  To Workspace9 : ToWorkspace  VariableName=dXeff  SaveFormat=Timeseries  SampleTime=-1
  N : Outport
  wires:
  Bv/1 -> Selector10/1, Selector4/1, Selector8/1, Mz/2(Bv)
  Bx/1 -> Mz/1(Bx), Selector2/1
  Selector10/1 -> N'uvw/2, Product1/1  "speed"
  Ba/1 -> Mz/3(Ba)
  UeX/1 -> Mz/9(UeX)
  Beta/1 -> Sign1/1, Abs2/1, To Workspace2/1
  Umag/1 -> Mz/8(Umag)
  dLCG/1 -> Mz/10(dLCG)
  dmass/1 -> Mz/11(dmass)
  dX/1 -> Scope4/1, To Workspace9/1, NdXi/1(dX)
  N'r/1 -> Product/2
  N'r|r|/1 -> Product6/2
  Product4/1 -> Abs3/1
  Selector8/1 -> Product4/1
  Selector4/1 -> Product1/2, Sign2/1, Product4/2, Product5/2, Product5/1, Sign3/1
  Product5/1 -> Abs/1
  Product3/1 -> Gain4/1
  Mz/1(N) -> Scope/1, N/1, Mux/6  "N Total"
  Selector2/1 -> NdXi/2(z), Saturation4/1  "z"
  N'uvw/1 -> Product2/2
  Product1/1 -> Sign/1, Abs1/1
  Abs1/1 -> N'r/1
  Sign/1 -> Product/1
  Product/1 -> Gain2/1
  Abs2/1 -> Scope2/1, N'uvw/1  "beta"
  Sign1/1 -> Product2/1
  Product2/1 -> Gain/1
  Gain/1 -> Mz/7(CNuvw)
  NdXi/1(NdXi) -> Gain1/1
  Gain1/1 -> Scope3/1, Mz/12(CNdXi)
  Nvm/1 -> Mux/5, Mz/13(Nvm)
  Mz/2(NApp) -> Mux/1  "N App"
  Mz/3(N_hull) -> Scope5/1, Mux/2  "N Hull"
  Mz/4(Nh_Total) -> Mux/3
  Mz/5(Nprop) -> Mux/4
  Mux/1 -> To Workspace8/1
  Mz/7(NAppAll) -> To Workspace1/1  "N"
  BFM/1 -> Selector1/1
  Selector1/1 -> Mz/14(BFN)
  [N_Stat] -> Mux/7
  Mz/6(NStat) -> [N_Stat]
  Gain2/1 -> Mz/4(CNr)
  Gain3/1 -> Mz/5(CNrr)
  Gain4/1 -> Mz/6(CNvr)
  Saturation4/1 -> N'uvw/3  "z"
  Mz/8(NHullVM) -> To Workspace3/1  "N_hull"
  Abs3/1 -> N'vr/1
  N'vr/1 -> Product3/1
  Sign2/1 -> Product3/2
  Product6/1 -> Gain3/1
  Sign3/1 -> Product6/1
  Mz/9(Nvr) -> Scope5/5, To Workspace4/1  "Nvr"
  Mz/10(Nrr) -> Scope5/4, To Workspace5/1  "Nrr"
  Mz/11(Nuvw) -> To Workspace6/1, Scope5/2  "Nuvw"
  Abs/1 -> N'r|r|/1
  Mz/12(Nr) -> To Workspace7/1, Scope5/3  "Nr"
